simulink model "ROBOT_DYNAMICS"  (R2024a)
settings: Solver=ode5  StartTime=0.0  StopTime=10  FixedStep=1e-1  RelTol=1e-3
PreLoadFcn:
  | track_map = track_map;
values from neighbouring files (symbols this model uses):
  L = 10e-2    (= 0.1)    [LINE_CONTROL_SETUP.m]    (also in x_opt.mat)
  r = 3.5e-2    (= 0.035)    [LINE_CONTROL_SETUP.m]    (also in x_opt.mat)
  theta_0 = deg2rad(0)    [LINE_CONTROL_SETUP.m]    (also in x_opt.mat = 0)
  x0 = 1    [LINE_CONTROL_SETUP.m]    (also in x_opt.mat)
  y0 = 1.146    [LINE_CONTROL_SETUP.m]    (also in x_opt.mat)
settings Model: ParamWorkspaceSource=ReferencedWorkspace  Creator=pedro  LastModifiedBy=pedro

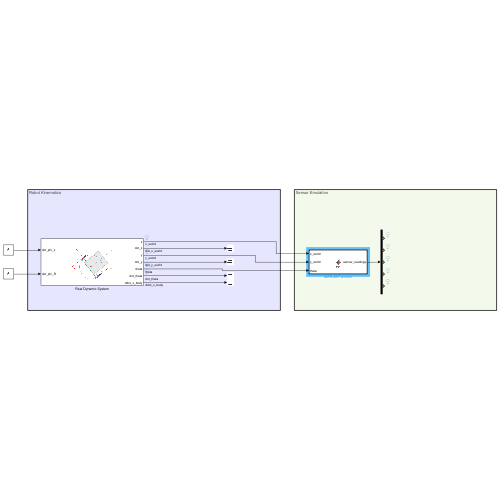
[thumbnail: Simulink's stored preview of the top-level diagram]
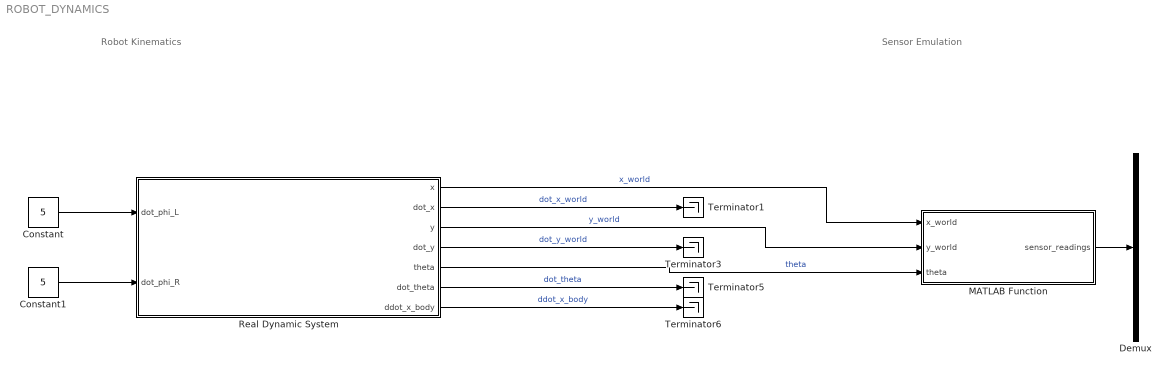
== system ROBOT_DYNAMICS ==
  note: Sensor Emulation
  note: Robot Kinematics
  Constant : Constant  Value=5
  Constant1 : Constant  Value=5
  Demux : Demux  Outputs=5
  MATLAB Function : MATLAB Function  TreatAsAtomicUnit=on
  Real Dynamic System : Subsystem
      mask Display: image('robot_model.png', [0,0,0,0,90,90]);
  Terminator{1,3,5..6} (4 alike) : Terminator
  wires:
  Real Dynamic System/1(x) -> MATLAB Function/1(x_world)  "x_world"
  Real Dynamic System/2(dot_x) -> Terminator1/1  "dot_x_world"
  Real Dynamic System/3(y) -> MATLAB Function/2(y_world)  "y_world"
  Real Dynamic System/4(dot_y) -> Terminator3/1  "dot_y_world"
  Real Dynamic System/5(theta) -> MATLAB Function/3(theta)  "theta"
  Real Dynamic System/6(dot_theta) -> Terminator5/1  "dot_theta"
  Real Dynamic System/7(ddot_x_body) -> Terminator6/1  "ddot_x_body"
  MATLAB Function/1(sensor_readings) -> Demux/1
  Constant/1 -> Real Dynamic System/1(dot_phi_L)
  Constant1/1 -> Real Dynamic System/2(dot_phi_R)

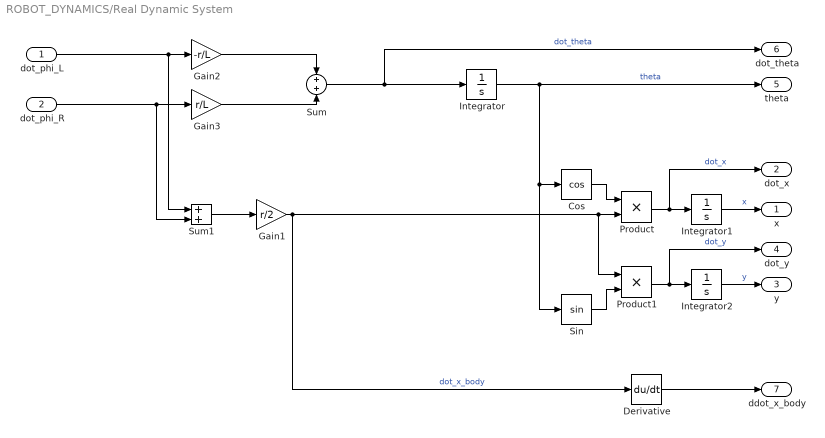
== system ROBOT_DYNAMICS/Real Dynamic System ==
  dot_phi_L : Inport
  dot_phi_R : Inport  Port=2
  Cos : Trigonometry  Operator=cos
  Derivative : Derivative
  Gain1 : Gain  Gain=r/2
  Gain2 : Gain  Gain=-r/L
  Gain3 : Gain  Gain=r/L
  Integrator : Integrator  InitialCondition=theta_0
  Integrator1 : Integrator  InitialCondition=x0
  Integrator2 : Integrator  InitialCondition=y0
  Product : Product
  Product1 : Product
  Sin : Trigonometry
  Sum : Sum  Inputs=+|+
  Sum1 : Sum
  x : Outport
  dot_x : Outport  Port=2
  y : Outport  Port=3
  dot_y : Outport  Port=4
  theta : Outport  Port=5
  dot_theta : Outport  Port=6
  ddot_x_body : Outport  Port=7
  wires:
  dot_phi_L/1 -> Sum1/1, Gain2/1
  Product1/1 -> dot_y/1, Integrator2/1  "dot_y"
  Cos/1 -> Product/1
  Integrator/1 -> theta/1, Sin/1, Cos/1  "theta"
  Gain3/1 -> Sum/2
  Product/1 -> dot_x/1, Integrator1/1  "dot_x"
  Gain1/1 -> Derivative/1, Product1/1, Product/2  "dot_x_body"
  Sum1/1 -> Gain1/1
  dot_phi_R/1 -> Sum1/2, Gain3/1
  Gain2/1 -> Sum/1
  Sum/1 -> dot_theta/1, Integrator/1  "dot_theta"
  Integrator1/1 -> x/1  "x"
  Integrator2/1 -> y/1  "y"
  Sin/1 -> Product1/2
  Derivative/1 -> ddot_x_body/1

== matlab function ROBOT_DYNAMICS/MATLAB Function ==
  data: x_world input; sensor_readings output; y_world input; theta input; track_map parameter
function sensor_readings = fcn(x_world, y_world, theta, track_map)

theta = theta - pi/2;
rotation_matrix = [cos(theta) -sin(theta)
                    sin(theta) cos(theta)];

x_world = squeeze(x_world);
y_world = squeeze(y_world);
theta   = squeeze(theta);

P_sensor_1 = [5.5e-2  7e-2]';
P_sensor_2 = [3e-2    7e-2]';
P_sensor_3 = [0     8.5e-2]';
P_sensor_4 = [-3e-2   7e-2]';
P_sensor_5 = [-5.5e-2 7e-2]';

sensor_1_coord = [x_world y_world]' + rotation_matrix * P_sensor_1;
sensor_2_coord = [x_world y_world]' + rotation_matrix * P_sensor_2;
sensor_3_coord = [x_world y_world]' + rotation_matrix * P_sensor_3;
sensor_4_coord = [x_world y_world]' + rotation_matrix * P_sensor_4;
sensor_5_coord = [x_world y_world]' + rotation_matrix * P_sensor_5;

sensor_1_coord = ceil(sensor_1_coord*1e3); % Convert to mm since 1px=1mm
sensor_2_coord = ceil(sensor_2_coord*1e3); % Convert to mm since 1px=1mm
sensor_3_coord = ceil(sensor_3_coord*1e3); % Convert to mm since 1px=1mm
sensor_4_coord = ceil(sensor_4_coord*1e3); % Convert to mm since 1px=1mm
sensor_5_coord = ceil(sensor_5_coord*1e3); % Convert to mm since 1px=1mm

%max_line_sensor_value = 2500;
%min_line_sensor_value = 500;

track_index_size = flip(size(track_map));
sensor_readings = zeros(1, 5);

if any(track_index_size' < [sensor_1_coord sensor_2_coord sensor_3_coord sensor_4_coord sensor_5_coord], 'all') || any([0;0] >= [sensor_1_coord sensor_2_coord sensor_3_coord sensor_4_coord sensor_5_coord], 'all')
    %sensor_readings(sensor_readings == 0) = min_line_sensor_value;
    return
end

sensor_readings(1) = track_map(sensor_1_coord(2), sensor_1_coord(1));
sensor_readings(2) = track_map(sensor_2_coord(2), sensor_2_coord(1));
sensor_readings(3) = track_map(sensor_3_coord(2), sensor_3_coord(1));
sensor_readings(4) = track_map(sensor_4_coord(2), sensor_4_coord(1));
sensor_readings(5) = track_map(sensor_5_coord(2), sensor_5_coord(1));

%sensor_readings(sensor_readings == 0)   = min_line_sensor_value;
%sensor_readings(sensor_readings == 1) = max_line_sensor_value;
